simulink model "WholeControlSystemWithQuantizationError"  (R2019a)
settings: Solver=ode4  StartTime=0.0  StopTime=50  FixedStep=1e-4  MaxStep=1e-4  MinStep=1e-8  RelTol=1e-10
InitFcn:
  | Rs = 0.011
  | Ld = 0.018
  | Lq = 0.018
  | Fi = 0.055
  | p = 4
  | J = 0.102
  | b = 0.18
  | 
  | A1 = 1
  | B1 = -5000
  | B2 = -0.0200
  | B3 = 10
  | C1 = 500
  | C2 = -2.499999800000000e+04
  | C3 = -90.999999999999990
  | C4 = 110
  | 
  | tC = 20
  | kk1 = -211
  | kk2 = -15
  | kk3 = -2.3
  | k3 = -1.586440829524976
  | k4 = -0.541242258944882
  | k5 = -0.541242258944882
  | k6 = -0.328094464592671
  | 
  | x1e = 0.001479483606571
  | x2e = 0
  | x3e = 0.739741803285525
  | ide = 2.930555555555555
  | iqe = 0.605243293597248
  | 
  | g1 = 0.164052784000000
  | g2 = -2.996000000000000
  | g3 = 8.089800000000000e+02
  | 
  | h1=1e-4*80
libraries: simulink x1
settings Model: Creator=LiLid  LastModifiedBy=LiLid

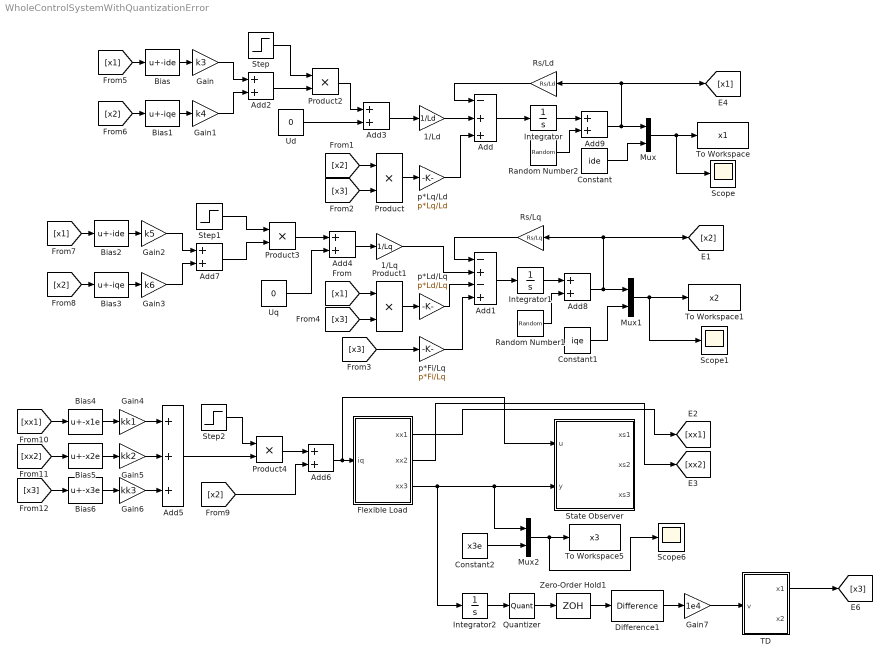
== system WholeControlSystemWithQuantizationError ==
  1/Ld : Gain  Gain=1/Ld
  1/Lq : Gain  Gain=1/Lq
  Add : Sum  Inputs=-++
  Add1 : Sum  Inputs=-+-+
  Add{2..4,6..9} (7 alike) : Sum
  Add5 : Sum  Inputs=+++
  Bias : Bias  Bias=-ide
  Bias1 : Bias  Bias=-iqe
  Bias2 : Bias  Bias=-ide
  Bias3 : Bias  Bias=-iqe
  Bias4 : Bias  Bias=-x1e
  Bias5 : Bias  Bias=-x2e
  Bias6 : Bias  Bias=-x3e
  Constant : Constant  Value=ide
  Constant1 : Constant  Value=iqe
  Constant2 : Constant  Value=x3e
  Difference1 : simulink/Discrete/Difference  ICPrevInput=0.0  OutMin=[]  OutMax=[]  OutDataType=fixdt(1, 16)  OutScaling=2^-10  DoSatur=off
  Flexible Load : Subsystem
  Gain : Gain  Gain=k3
  Gain1 : Gain  Gain=k4
  Gain2 : Gain  Gain=k5
  Gain3 : Gain  Gain=k6
  Gain4 : Gain  Gain=kk1
  Gain5 : Gain  Gain=kk2
  Gain6 : Gain  Gain=kk3
  Gain7 : Gain  Gain=1e4
  Integrator : Integrator  InitialCondition=0.15
  Integrator1 : Integrator  InitialCondition=0.14
  Integrator2 : Integrator
  Mux : Mux  Inputs=2
  Mux1 : Mux  Inputs=2
  Mux2 : Mux  Inputs=2
  Product{,1..4} (5 alike) : Product
  Quantizer : Quantizer  QuantizationInterval=2*pi/31488
  Random Number1 : RandomNumber  Variance=0  SampleTime=0.0005
  Random Number2 : RandomNumber  Variance=0  SampleTime=0.0005
  Rs/Ld : Gain  Gain=Rs/Ld
  Rs/Lq : Gain  Gain=Rs/Lq
  Scope : Scope
  Scope1 : Scope
  Scope6 : Scope
  State Observer : Subsystem
  Step : Step  Time=tC  SampleTime=0
  Step1 : Step  Time=tC  SampleTime=0
  Step2 : Step  Time=tC  SampleTime=0
  TD : Subsystem
  To Workspace : ToWorkspace  VariableName=x1  SampleTime=-1
      settings: Save2DSignal=2-D array (concatenate along first dimension)
  To Workspace1 : ToWorkspace  VariableName=x2  SampleTime=-1
      settings: Save2DSignal=2-D array (concatenate along first dimension)
  To Workspace5 : ToWorkspace  VariableName=x3  SampleTime=-1
      settings: Save2DSignal=2-D array (concatenate along first dimension)
  Ud : Constant  Value=0
  Uq : Constant  Value=0
  Zero-Order Hold1 : ZeroOrderHold  SampleTime=1e-4
  p*Fi/Lq : Gain  Gain=p*Fi/Lq
  p*Ld/Lq : Gain  Gain=p*Ld/Lq
  p*Lq/Ld : Gain  Gain=p*Lq/Ld
  wires:
  Add/1 -> Integrator/1
  Rs/Ld/1 -> Add/1
  Product/1 -> p*Lq/Ld/1
  [x2] -> Product/1
  [x3] -> Product/2
  Rs/Lq/1 -> Add1/1
  Add1/1 -> Integrator1/1
  [x1] -> Product1/1
  [x3] -> Product1/2
  [x3] -> p*Fi/Lq/1
  p*Fi/Lq/1 -> Add1/4
  p*Lq/Ld/1 -> Add/3
  1/Ld/1 -> Add/2
  1/Lq/1 -> Add1/2
  Product1/1 -> p*Ld/Lq/1
  p*Ld/Lq/1 -> Add1/3
  Gain1/1 -> Add2/2
  Gain/1 -> Add2/1
  Add2/1 -> Product2/2
  Ud/1 -> Add3/2
  Add3/1 -> 1/Ld/1
  Step/1 -> Product2/1
  Product2/1 -> Add3/1
  Add4/1 -> 1/Lq/1
  Uq/1 -> Add4/2
  Product3/1 -> Add4/1
  Bias/1 -> Gain/1
  Bias1/1 -> Gain1/1
  Gain2/1 -> Add7/1
  Bias2/1 -> Gain2/1
  Gain3/1 -> Add7/2
  Add7/1 -> Product3/2
  Step1/1 -> Product3/1
  Flexible Load/3(xx3) -> Integrator2/1, Mux2/1, State Observer/2(y)
  [x1] -> Bias/1
  [x2] -> Bias1/1
  [x1] -> Bias2/1
  Bias3/1 -> Gain3/1
  [x2] -> Bias3/1
  [xx1] -> Bias4/1
  [xx2] -> Bias5/1
  [x3] -> Bias6/1
  Bias4/1 -> Gain4/1
  Bias5/1 -> Gain5/1
  Bias6/1 -> Gain6/1
  Gain4/1 -> Add5/1
  Gain5/1 -> Add5/2
  Gain6/1 -> Add5/3
  Add5/1 -> Product4/2
  Step2/1 -> Product4/1
  Product4/1 -> Add6/1
  [x2] -> Add6/2
  Add6/1 -> State Observer/1(u), Flexible Load/1(iq)
  Mux/1 -> Scope/1, To Workspace/1
  Constant/1 -> Mux/2
  Constant1/1 -> Mux1/2
  Mux1/1 -> To Workspace1/1, Scope1/1
  Constant2/1 -> Mux2/2
  Mux2/1 -> Scope6/1, To Workspace5/1
  Flexible Load/1(xx1) -> [xx1]
  Flexible Load/2(xx2) -> [xx2]
  Integrator2/1 -> Quantizer/1
  Quantizer/1 -> Zero-Order Hold1/1
  Zero-Order Hold1/1 -> Difference1/1
  Difference1/1 -> Gain7/1
  Gain7/1 -> TD/1(v)
  TD/1(x1) -> [x3]
  Integrator1/1 -> Add8/1
  Random Number1/1 -> Add8/2
  Add8/1 -> Rs/Lq/1, [x2], Mux1/1
  Random Number2/1 -> Add9/2
  Integrator/1 -> Add9/1
  Add9/1 -> [x1], Rs/Ld/1, Mux/1

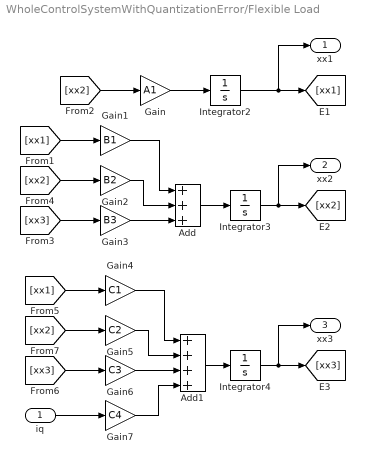
== system WholeControlSystemWithQuantizationError/Flexible Load ==
  iq : Inport
  Add : Sum  Inputs=+++
  Add1 : Sum  Inputs=++++
  Gain : Gain  Gain=A1
  Gain1 : Gain  Gain=B1
  Gain2 : Gain  Gain=B2
  Gain3 : Gain  Gain=B3
  Gain4 : Gain  Gain=C1
  Gain5 : Gain  Gain=C2
  Gain6 : Gain  Gain=C3
  Gain7 : Gain  Gain=C4
  Integrator2 : Integrator
  Integrator3 : Integrator
  Integrator4 : Integrator
  xx1 : Outport
  xx2 : Outport  Port=2
  xx3 : Outport  Port=3
  wires:
  Integrator2/1 -> xx1/1, [xx1]
  Integrator3/1 -> [xx2], xx2/1
  Integrator4/1 -> xx3/1, [xx3]
  [xx2] -> Gain/1
  Gain/1 -> Integrator2/1
  [xx1] -> Gain1/1
  [xx2] -> Gain2/1
  [xx3] -> Gain3/1
  Add/1 -> Integrator3/1
  Gain3/1 -> Add/3
  Gain2/1 -> Add/2
  Gain1/1 -> Add/1
  [xx1] -> Gain4/1
  [xx2] -> Gain5/1
  Add1/1 -> Integrator4/1
  Gain5/1 -> Add1/2
  [xx3] -> Gain6/1
  Gain6/1 -> Add1/3
  Gain4/1 -> Add1/1
  iq/1 -> Gain7/1
  Gain7/1 -> Add1/4

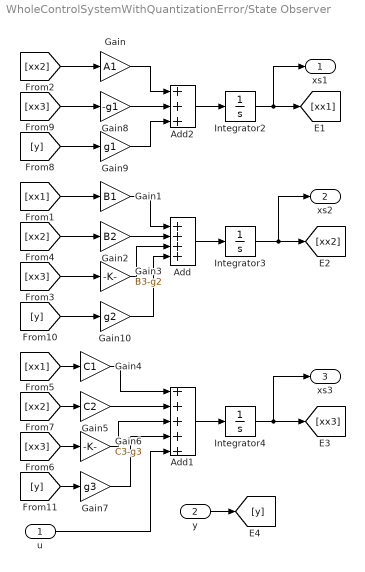
== system WholeControlSystemWithQuantizationError/State Observer ==
  u : Inport
  y : Inport  Port=2
  Add : Sum  Inputs=++++
  Add1 : Sum  Inputs=+++++
  Add2 : Sum  Inputs=+++
  Gain : Gain  Gain=A1
  Gain1 : Gain  Gain=B1
  Gain10 : Gain  Gain=g2
  Gain2 : Gain  Gain=B2
  Gain3 : Gain  Gain=B3-g2
  Gain4 : Gain  Gain=C1
  Gain5 : Gain  Gain=C2
  Gain6 : Gain  Gain=C3-g3
  Gain7 : Gain  Gain=g3
  Gain8 : Gain  Gain=-g1
  Gain9 : Gain  Gain=g1
  Integrator2 : Integrator
  Integrator3 : Integrator
  Integrator4 : Integrator
  xs1 : Outport
  xs2 : Outport  Port=2
  xs3 : Outport  Port=3
  wires:
  Integrator3/1 -> [xx2], xs2/1
  Integrator4/1 -> [xx3], xs3/1
  [xx2] -> Gain/1
  [xx1] -> Gain1/1
  [xx2] -> Gain2/1
  [xx3] -> Gain3/1
  Add/1 -> Integrator3/1
  Gain3/1 -> Add/3
  Gain2/1 -> Add/2
  Gain1/1 -> Add/1
  [xx1] -> Gain4/1
  [xx2] -> Gain5/1
  Add1/1 -> Integrator4/1
  Gain5/1 -> Add1/2
  [xx3] -> Gain6/1
  Gain6/1 -> Add1/3
  Gain4/1 -> Add1/1
  Gain7/1 -> Add1/4
  y/1 -> [y]
  [xx3] -> Gain8/1
  [y] -> Gain9/1
  Gain8/1 -> Add2/2
  Gain9/1 -> Add2/3
  Gain/1 -> Add2/1
  Add2/1 -> Integrator2/1
  Integrator2/1 -> xs1/1, [xx1]
  Gain10/1 -> Add/4
  [y] -> Gain10/1
  [y] -> Gain7/1
  u/1 -> Add1/5

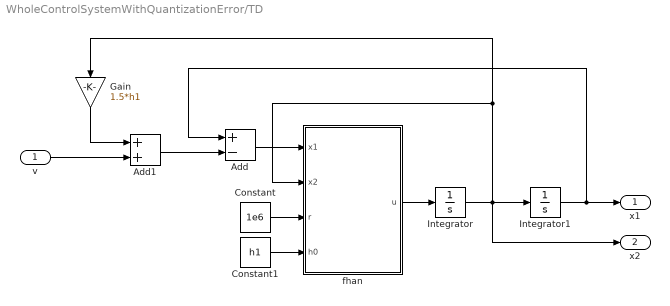
== system WholeControlSystemWithQuantizationError/TD ==
  v : Inport
  Add : Sum  Inputs=+-
  Add1 : Sum
  Constant : Constant  Value=1e6
  Constant1 : Constant  Value=h1
  Gain : Gain  Gain=1.5*h1
  Integrator : Integrator
  Integrator1 : Integrator
  fhan : Subsystem
  x1 : Outport
  x2 : Outport  Port=2
  wires:
  fhan/1(u) -> Integrator/1
  Integrator/1 -> x2/1, fhan/2(x2), Gain/1, Integrator1/1
  Integrator1/1 -> x1/1, Add/1
  Add/1 -> fhan/1(x1)
  Constant/1 -> fhan/3(r)
  Constant1/1 -> fhan/4(h0)
  Add1/1 -> Add/2
  Gain/1 -> Add1/1
  v/1 -> Add1/2

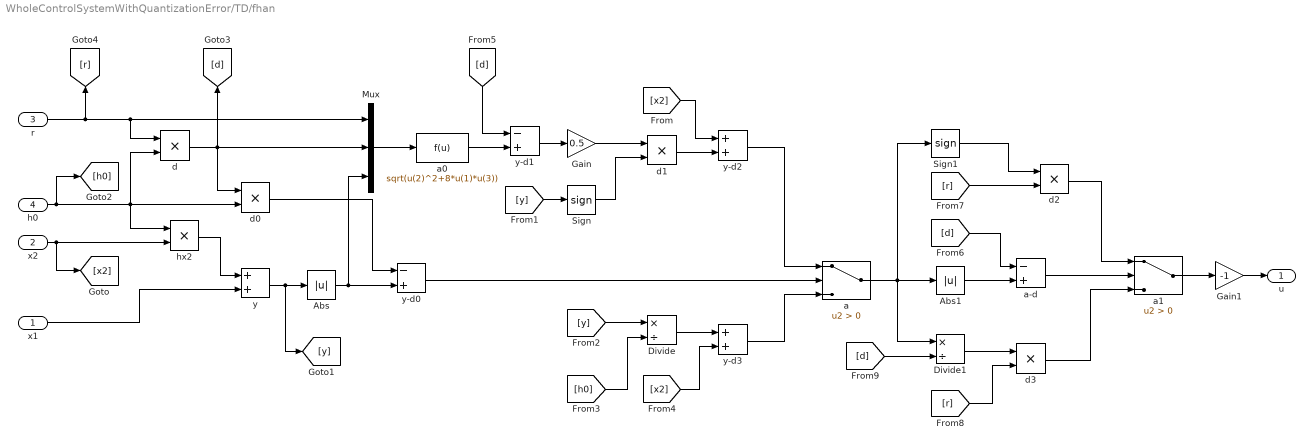
== system WholeControlSystemWithQuantizationError/TD/fhan ==
  x1 : Inport
  x2 : Inport  Port=2
  r : Inport  Port=3
  h0 : Inport  Port=4
  Abs : Abs
  Abs1 : Abs
  Divide : Product  Inputs=*/
  Divide1 : Product  Inputs=*/
  Gain : Gain  Gain=0.5
  Gain1 : Gain  Gain=-1
  Mux : Mux  Inputs=3
  Sign : Signum
  Sign1 : Signum
  a : Switch  Criteria=u2 > Threshold
  a-d : Sum  Inputs=-+
  a0 : Fcn  Expr=sqrt(u(2)^2+8*u(1)*u(3))
  a1 : Switch  Criteria=u2 > Threshold
  d{,0..3} (5 alike) : Product
  hx2 : Product
  y : Sum
  y-d0 : Sum  Inputs=-+
  y-d1 : Sum  Inputs=-+
  y-d2 : Sum
  y-d3 : Sum
  u : Outport
  wires:
  h0/1 -> [h0], d/2, hx2/1, d0/2
  r/1 -> [r], d/1, Mux/1
  d/1 -> d0/1, [d], Mux/2
  x2/1 -> hx2/2, [x2]
  x1/1 -> y/2
  hx2/1 -> y/1
  Mux/1 -> a0/1
  y/1 -> [y], Abs/1
  Abs/1 -> y-d0/2, Mux/3
  d0/1 -> y-d0/1
  y-d0/1 -> a/2
  a0/1 -> y-d1/2
  y-d1/1 -> Gain/1
  Gain/1 -> d1/1
  Sign/1 -> d1/2
  d1/1 -> y-d2/2
  [x2] -> y-d2/1
  [y] -> Sign/1
  y-d2/1 -> a/1
  [y] -> Divide/1
  [h0] -> Divide/2
  Divide/1 -> y-d3/1
  [x2] -> y-d3/2
  y-d3/1 -> a/3
  a/1 -> Divide1/1, Sign1/1, Abs1/1
  Abs1/1 -> a-d/2
  [d] -> y-d1/1
  [d] -> a-d/1
  a-d/1 -> a1/2
  [r] -> d2/2
  Sign1/1 -> d2/1
  d2/1 -> a1/1
  [d] -> Divide1/2
  Divide1/1 -> d3/1
  [r] -> d3/2
  d3/1 -> a1/3
  a1/1 -> Gain1/1
  Gain1/1 -> u/1
